simulink subsystem "Long_Vert_Aero_Forces_Moments"  (R2025b)
settings: Solver=VariableStepAuto  StartTime=0.0  StopTime=10.0  RelTol=1e-3
undefined symbols (not defined in the file): alpha, Cbar, CD0, CD_alpha, CD_delEle, CD_ih, CD_row, CL0, CL_alpha, CL_delEle, CL_ih, CL_row, CM0, CM_alpha, CM_delEle, CM_ih, CM_row, Sref, u0
libraries: simulink_extras x2
settings Model: Creator=cdriggs  LastModifiedBy=cdriggs

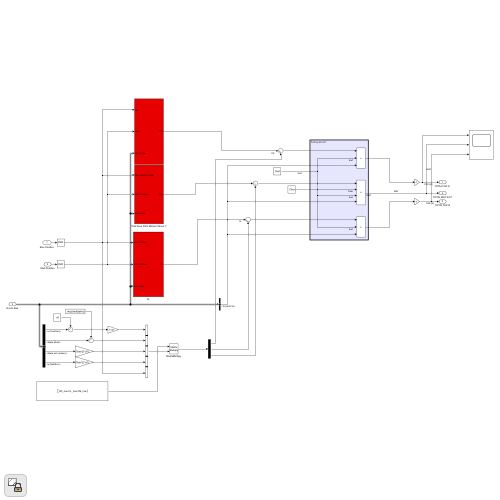
[thumbnail: Simulink's stored preview of the top-level diagram]
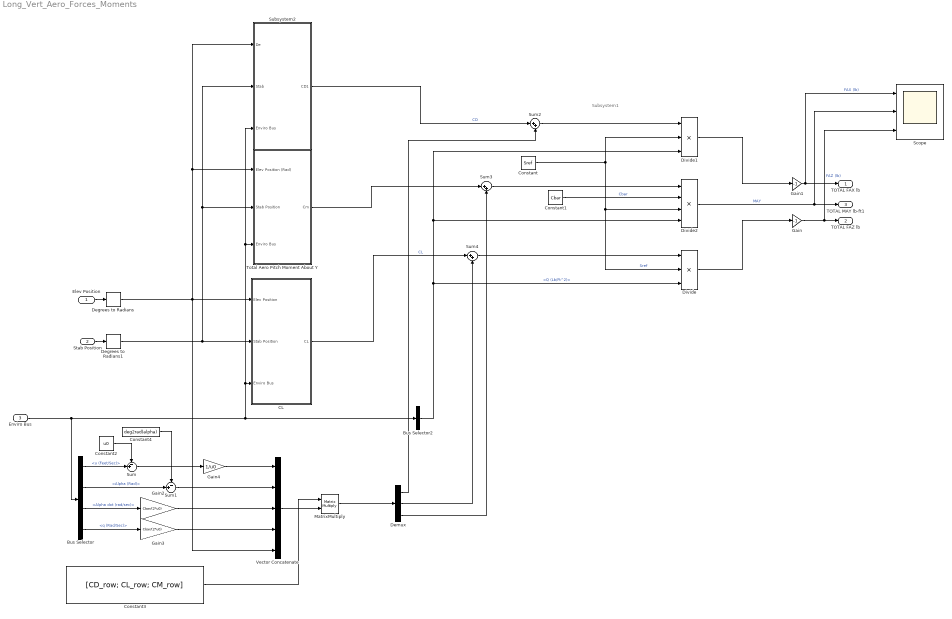
== system Long_Vert_Aero_Forces_Moments ==
  note: Subsystem1
  Elev Position : Inport
  Stab Position : Inport  Port=2
  Enviro Bus : Inport  Port=3
  Bus Selector : BusSelector  OutputSignals=Trans.Body Veloc.u (Feet/Sec),Aero angles.Alpha (Rad),Aero angles.Alpha dot (rad/sec),Rotat.Body.Rates (Rad/Sec).q (Rad/Sec)
  Bus Selector2 : BusSelector  OutputSignals=Q (Lb/Ft^2)
  CL : Subsystem
  Constant : Constant  Value=Sref
  Constant1 : Constant  Value=Cbar
  Constant2 : Constant  Value=u0
  Constant3 : Constant  Value=[CD_row; CL_row; CM_row]
  Constant4 : Constant  Value=deg2rad(alpha)
  Degrees to Radians : simulink_extras/Transformations/Degrees to Radians
  Degrees to Radians1 : simulink_extras/Transformations/Degrees to Radians
  Demux : Demux  Outputs=3
  Divide : Product  Inputs=***
  Divide1 : Product  Inputs=***
  Divide2 : Product  Inputs=****
  Gain : Gain  Gain=-1
  Gain1 : Gain  Gain=-1
  Gain2 : Gain  Gain=Cbar/(2*u0)
  Gain3 : Gain  Gain=Cbar/(2*u0)
  Gain4 : Gain  Gain=1/u0
  MatrixMultiply : Product  Multiplication=Matrix(*)
  Scope : Scope  NumInputPorts=3
      settings: ActiveDisplayYMinimum=-64560.4205403159  ActiveDisplayYMaximum=-64554.93444293263  DataLoggingVariableName=ScopeData7
  Subsystem2 : Subsystem
  Sum : Sum  Inputs=-+|
  Sum1 : Sum  Inputs=-+|
  Sum2 : Sum  Inputs=|++
  Sum3 : Sum  Inputs=|++
  Sum4 : Sum  Inputs=|++
  Total Aero Pitch Moment About Y : Subsystem
  Vector Concatenate : Concatenate  NumInputs=5
  "TOTAL FAX lb " : Outport
  TOTAL FAZ lb : Outport  Port=2
  TOTAL MAY lb-ft1 : Outport  Port=3
  wires:
  Degrees to Radians1/1 -> CL/2(Stab Position), Total Aero Pitch Moment About Y/2(Stab Position), Subsystem2/2(Stab)
  Divide2/1 -> Scope/2, TOTAL MAY lb-ft1/1  "MAY"
  Stab Position/1 -> Degrees to Radians1/1
  Enviro Bus/1 -> Bus Selector2/1, CL/3(Enviro Bus), Subsystem2/3(Enviro Bus), Total Aero Pitch Moment About Y/3(Enviro Bus), Bus Selector/1
  Degrees to Radians/1 -> CL/1(Elev Position), Total Aero Pitch Moment About Y/1(Elev Position (Rad)), Subsystem2/1(De), Vector Concatenate/5
  Constant/1 -> Divide1/2, Divide/2, Divide2/3  "Sref"
  Gain/1 -> TOTAL FAZ lb/1, Scope/3  "FAZ (lb)"
  Divide1/1 -> Gain1/1
  Constant1/1 -> Divide2/2  "Cbar"
  Subsystem2/1(CD1) -> Sum2/1  "CD"
  Gain1/1 -> "TOTAL FAX lb "/1, Scope/1  "FAX (lb)"
  CL/1(CL) -> Sum4/1  "CL"
  Bus Selector2/1 -> Divide1/3, Divide2/4, Divide/3  "<Q (Lb/Ft^2)>"
  Divide/1 -> Gain/1
  Elev Position/1 -> Degrees to Radians/1
  Total Aero Pitch Moment About Y/1(Cm) -> Sum3/1
  Bus Selector/1 -> Sum/2  "<u (Feet/Sec)>"
  Bus Selector/2 -> Sum1/2  "<Alpha (Rad)>"
  Bus Selector/3 -> Gain2/1  "<Alpha dot (rad/sec)>"
  Bus Selector/4 -> Gain3/1  "<q (Rad/Sec)>"
  Constant2/1 -> Sum/1
  Gain2/1 -> Vector Concatenate/3
  Gain3/1 -> Vector Concatenate/4
  Constant4/1 -> Sum1/1
  Sum1/1 -> Vector Concatenate/2
  Vector Concatenate/1 -> MatrixMultiply/2
  Sum2/1 -> Divide1/1
  Sum3/1 -> Divide2/1
  Sum4/1 -> Divide/1
  Demux/1 -> Sum2/2
  Demux/2 -> Sum4/2
  Demux/3 -> Sum3/2
  Gain4/1 -> Vector Concatenate/1
  Sum/1 -> Gain4/1
  MatrixMultiply/1 -> Demux/1
  Constant3/1 -> MatrixMultiply/1

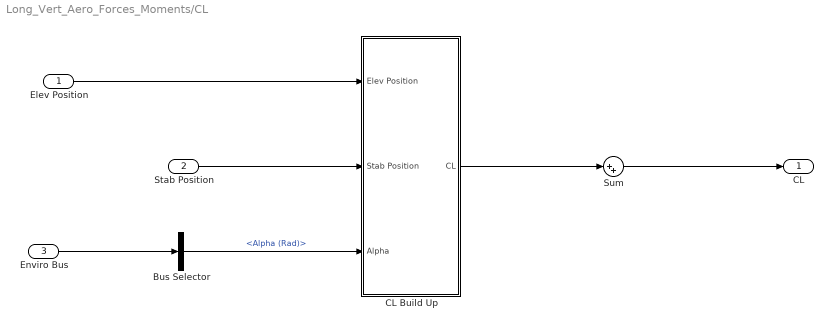
== system Long_Vert_Aero_Forces_Moments/CL ==
  Elev Position : Inport
  Stab Position : Inport  Port=2
  Enviro Bus : Inport  Port=3
  Bus Selector : BusSelector  OutputSignals=Aero angles.Alpha (Rad)
  CL Build Up : Subsystem
  Sum : Sum  Inputs=|++
  CL : Outport
  wires:
  Sum/1 -> CL/1
  CL Build Up/1(CL) -> Sum/1
  Enviro Bus/1 -> Bus Selector/1
  Bus Selector/1 -> CL Build Up/3(Alpha)  "<Alpha (Rad)>"
  Stab Position/1 -> CL Build Up/2(Stab Position)
  Elev Position/1 -> CL Build Up/1(Elev Position)

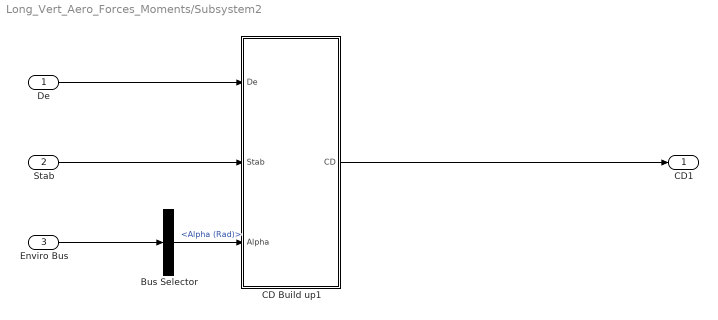
== system Long_Vert_Aero_Forces_Moments/Subsystem2 ==
  De : Inport
  Stab : Inport  Port=2
  Enviro Bus : Inport  Port=3
  Bus Selector : BusSelector  OutputSignals=Aero angles.Alpha (Rad)
  CD Build up1 : Subsystem
  CD1 : Outport
  wires:
  Bus Selector/1 -> CD Build up1/3(Alpha)  "<Alpha (Rad)>"
  Enviro Bus/1 -> Bus Selector/1
  CD Build up1/1(CD) -> CD1/1
  De/1 -> CD Build up1/1(De)
  Stab/1 -> CD Build up1/2(Stab)

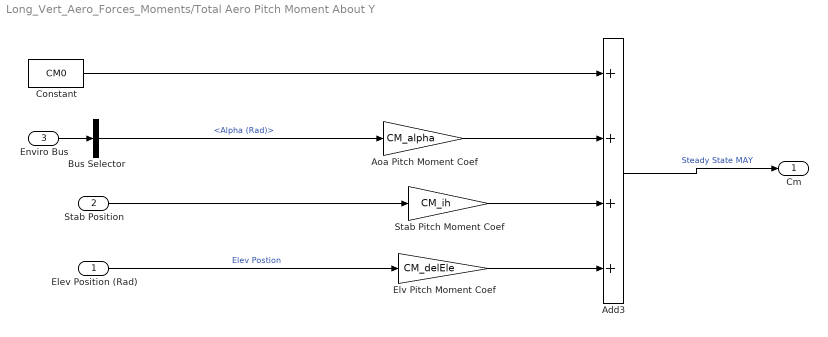
== system Long_Vert_Aero_Forces_Moments/Total Aero Pitch Moment About Y ==
  Elev Position (Rad) : Inport
  Stab Position : Inport  Port=2
  Enviro Bus : Inport  Port=3
  Add3 : Sum  Inputs=++++
  Aoa Pitch Moment Coef : Gain  Gain=CM_alpha
  Bus Selector : BusSelector  OutputSignals=Aero angles.Alpha (Rad)
  Constant : Constant  Value=CM0
  Elv Pitch Moment Coef : Gain  Gain=CM_delEle
  Stab Pitch Moment Coef : Gain  Gain=CM_ih
  Cm : Outport
  wires:
  Constant/1 -> Add3/1
  Elv Pitch Moment Coef/1 -> Add3/4
  Stab Pitch Moment Coef/1 -> Add3/3
  Stab Position/1 -> Stab Pitch Moment Coef/1
  Aoa Pitch Moment Coef/1 -> Add3/2
  Add3/1 -> Cm/1  "Steady State MAY"
  Enviro Bus/1 -> Bus Selector/1
  Elev Position (Rad)/1 -> Elv Pitch Moment Coef/1  "Elev Postion"
  Bus Selector/1 -> Aoa Pitch Moment Coef/1  "<Alpha (Rad)>"

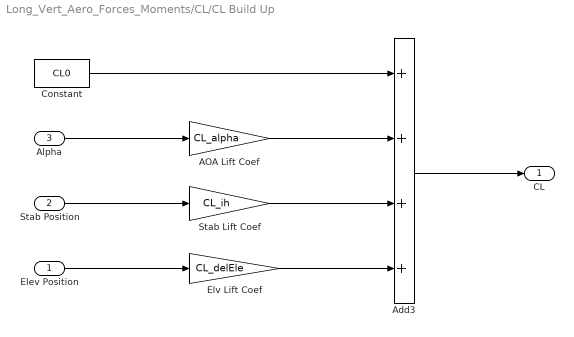
== system Long_Vert_Aero_Forces_Moments/CL/CL Build Up ==
  Elev Position : Inport
  Stab Position : Inport  Port=2
  Alpha : Inport  Port=3
  AOA Lift Coef : Gain  Gain=CL_alpha
  Add3 : Sum  Inputs=++++
  Constant : Constant  Value=CL0
  Elv Lift Coef : Gain  Gain=CL_delEle
  Stab Lift Coef : Gain  Gain=CL_ih
  CL : Outport
  wires:
  Alpha/1 -> AOA Lift Coef/1
  Elv Lift Coef/1 -> Add3/4
  AOA Lift Coef/1 -> Add3/2
  Stab Lift Coef/1 -> Add3/3
  Stab Position/1 -> Stab Lift Coef/1
  Add3/1 -> CL/1
  Elev Position/1 -> Elv Lift Coef/1
  Constant/1 -> Add3/1

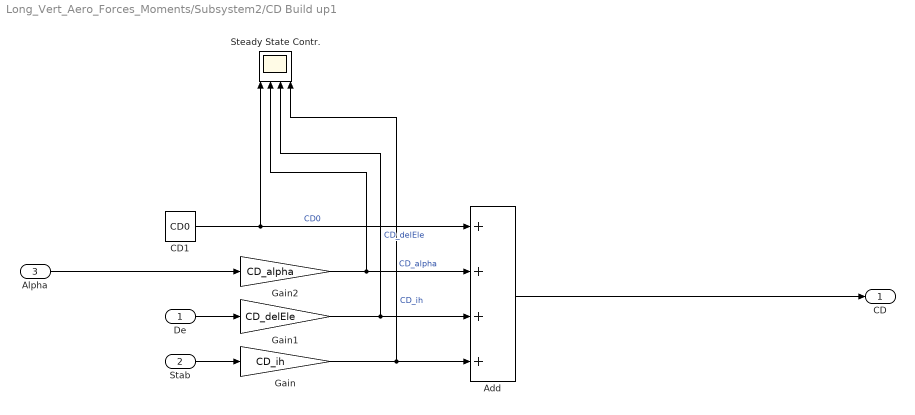
== system Long_Vert_Aero_Forces_Moments/Subsystem2/CD Build up1 ==
  De : Inport
  Stab : Inport  Port=2
  Alpha : Inport  Port=3
  Add : Sum  Inputs=++++
  CD1 : Constant  Value=CD0
  Gain : Gain  Gain=CD_ih
  Gain1 : Gain  Gain=CD_delEle
  Gain2 : Gain  Gain=CD_alpha
  Steady State Contr. : Scope  NumInputPorts=4
      settings: ActiveDisplayYMinimum=0.020499999999999997  ActiveDisplayYMaximum=0.0405  DataLoggingVariableName=ScopeData20
  CD : Outport
  wires:
  Gain1/1 -> Add/3, Steady State Contr./3  "CD_delEle"
  Gain2/1 -> Add/2, Steady State Contr./2  "CD_alpha"
  CD1/1 -> Add/1, Steady State Contr./1  "CD0"
  Add/1 -> CD/1
  De/1 -> Gain1/1
  Stab/1 -> Gain/1
  Gain/1 -> Steady State Contr./4, Add/4  "CD_ih"
  Alpha/1 -> Gain2/1
